simulink model "task5_lab14"  (R2021a)
settings: Solver=VariableStepAuto  StartTime=0.0  StopTime=10.0  RelTol=1e-3
settings Model: Creator=reemb  LastModifiedBy=reemb

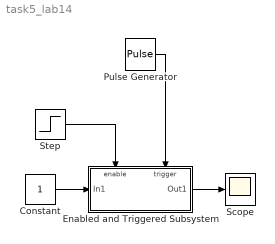
== system task5_lab14 ==
  Constant : Constant
  Enabled and Triggered Subsystem : Subsystem  TreatAsAtomicUnit=on
  Pulse Generator : DiscretePulseGenerator  PulseType=Time based  Period=1  PulseWidth=50
  Scope : Scope
  Step : Step  Time=5  SampleTime=0
  wires:
  Enabled and Triggered Subsystem/1(Out1) -> Scope/1
  Step/1 -> Enabled and Triggered Subsystem/Enable
  Constant/1 -> Enabled and Triggered Subsystem/1(In1)
  Pulse Generator/1 -> Enabled and Triggered Subsystem/Trigger

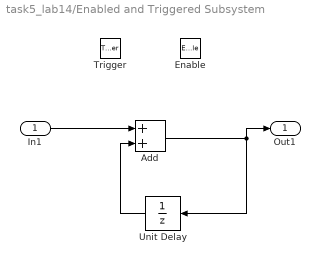
== system task5_lab14/Enabled and Triggered Subsystem ==
  In1 : Inport
  Enable : EnablePort  StatesWhenEnabling=reset
  Trigger : TriggerPort  VariantControl=(inherit)
  Add : Sum
  Unit Delay : UnitDelay  SampleTime=-1  HasFrameUpgradeWarning=on
  Out1 : Outport  OutputWhenDisabled=reset
  wires:
  Add/1 -> Unit Delay/1, Out1/1
  In1/1 -> Add/1
  Unit Delay/1 -> Add/2
